simulink model "FPGA_TEST"  (R2023b)
settings: Solver=VariableStepAuto  StartTime=0.0  StopTime=10.0  RelTol=1e-3
libraries: hwlogicconnlib x2
settings Model: Creator=lenovo GAME  LastModifiedBy=lenovo GAME
settings OptimizationCC: BlockReduction=off  ConditionallyExecuteInputs=off  DefaultParameterBehavior=Inlined
settings DebuggingCC: AlgebraicLoopMsg=error
settings HardwareCC: ProdBitPerPointer=32  ProdBitPerSizeT=32  ProdBitPerPtrDiffT=32  ProdLargestAtomicFloat=None  ProdIntDivRoundTo=Undefined  ProdEndianess=Unspecified  ProdWordSize=32  ProdHWDeviceType=ASIC/FPGA->ASIC/FPGA  TargetBitPerPointer=64  TargetBitPerSizeT=64  TargetBitPerPtrDiffT=64  TargetLongLongMode=on  TargetIntDivRoundTo=Zero  TargetEndianess=LittleEndian  TargetWordSize=64  TargetHWDeviceType=Custom Processor->MATLAB Host Computer  ProdEqTarget=off

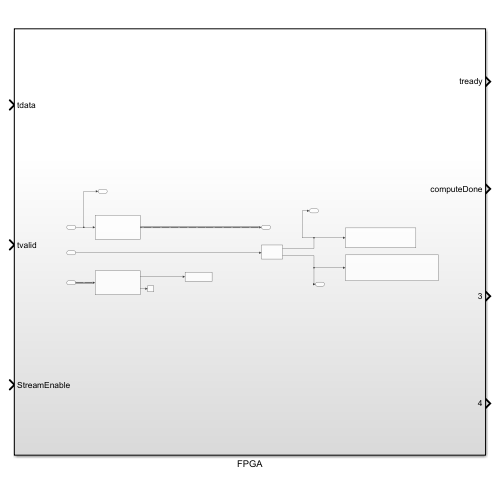
[thumbnail: Simulink's stored preview of the top-level diagram]
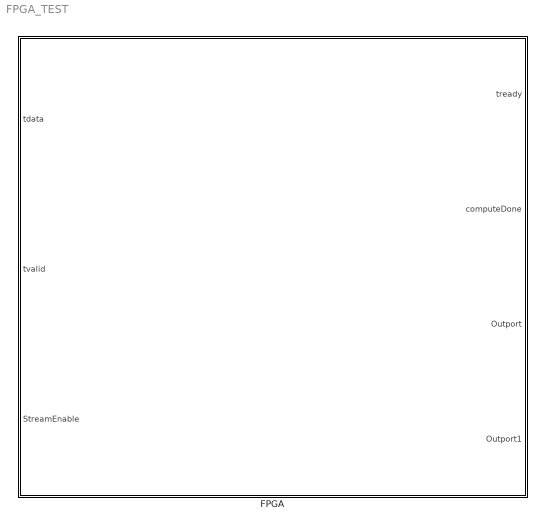
== system FPGA_TEST ==
  FPGA : Subsystem

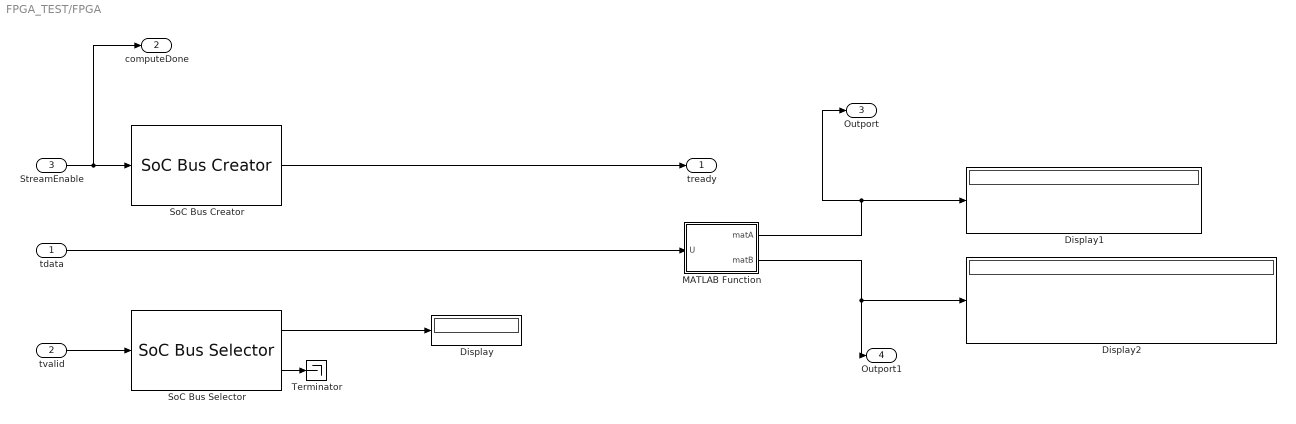
== system FPGA_TEST/FPGA ==
  tdata : Inport  OutDataTypeStr=double  PortDimensions=25
  tvalid : Inport  Port=2  OutDataTypeStr=Bus: StreamM2SBusObj
  StreamEnable : Inport  Port=3
  Display : Display
  Display1 : Display
  Display2 : Display
  MATLAB Function : MATLAB Function  TreatAsAtomicUnit=on
  SoC Bus Creator : hwlogicconnlib/SoC Bus Creator  Protocol=Data stream  ctrltype=Ready
  SoC Bus Selector : hwlogicconnlib/SoC Bus Selector  Protocol=Data stream  ctrltype=Valid
  Terminator : Terminator
  tready : Outport
  computeDone : Outport  Port=2
  Outport : Outport  Port=3
  Outport1 : Outport  Port=4
  wires:
  MATLAB Function/1(matA) -> Outport/1, Display1/1
  MATLAB Function/2(matB) -> Outport1/1, Display2/1
  tdata/1 -> MATLAB Function/1(U)
  SoC Bus Creator/1 -> tready/1
  StreamEnable/1 -> SoC Bus Creator/1, computeDone/1
  SoC Bus Selector/1 -> Display/1
  SoC Bus Selector/2 -> Terminator/1
  tvalid/1 -> SoC Bus Selector/1

== matlab function FPGA_TEST/FPGA/MATLAB Function ==
  data: U input; matA output; matB output
function [matA, matB] = fcn(U)   % U è 25x1 double
matA = reshape(U(1:9), [3 3]);
matB = reshape(U(10:25), [4 4]);
end
